simulink model "WDGBrakingLogic_Harness_SLDV"  (R2024a)
settings: Solver=FixedStepDiscrete  StartTime=0  StopTime=0.5  FixedStep=0.10000000000000001  RelTol=1e-3  EnableMultiTasking=on
Description:
  | Test harness for SLDV generated test cases.
settings Model: DataDictionary=DD_WDGBrakingLogic.sldd  EnableAccessToBaseWorkspace=off  Creator=The MathWorks, Inc.  LastModifiedBy=The MathWorks, Inc.
settings SolverCC: MaxZcPerStep=1
settings DataIOCC: LimitDataPoints=on
settings OptimizationCC: BlockReduction=off  DefaultParameterBehavior=Inlined  UseDivisionForNetSlopeComputation=on  GainParamInheritBuiltInType=on  UseFloatMulNetSlope=on  InlineInvariantSignals=on  ExpressionFolding=off  BitwiseOrLogicalOp=Bitwise operator  PassReuseOutputArgsAs=Individual arguments  InitFltsAndDblsToZero=on  EfficientFloat2IntCast=on  LifeSpan=inf  MaxStackSize=inf  OptimizeBlockOrder=speed  DifferentSizesBufferReuse=on  EfficientTunableParamExpr=on
settings DebuggingCC: SignalInfNanChecking=error  SignalRangeChecking=error  ReadBeforeWriteMsg=EnableAllAsError  WriteAfterWriteMsg=EnableAllAsError  WriteAfterReadMsg=EnableAllAsError  AlgebraicLoopMsg=error  ArtificialAlgebraicLoopMsg=error  SaveWithDisabledLinksMsg=error  SaveWithParameterizedLinksMsg=error  BlockPriorityViolationMsg=error  SolverPrmCheckMsg=error  InheritedTsInSrcMsg=none  SingleTaskRateTransMsg=error  TasksWithSamePriorityMsg=error  SigSpecEnsureSampleTimeMsg=error  CheckMatrixSingularityMsg=error  IntegerOverflowMsg=error  ParameterUnderflowMsg=error  ParameterPrecisionLossMsg=error  ParameterTunabilityLossMsg=error  UnderSpecifiedDataTypeMsg=error  UnnecessaryDatatypeConvMsg=warning  VectorMatrixConversionMsg=error  SignalLabelMismatchMsg=error  UnconnectedInputMsg=error  UnconnectedOutputMsg=error  UnconnectedLineMsg=error  SFcnCompatibilityMsg=error  UniqueDataStoreMsg=error  BusObjectLabelMismatch=error  RootOutportRequireBusObject=error  AssertControl=DisableAll  AllowSymbolicDim=off  ModelReferenceIOMismatchMessage=error  UnknownTsInhSupMsg=error  ModelReferenceDataLoggingMessage=error  ModelReferenceSymbolNameMessage=none  StateNameClashWarn=warning  PregeneratedLibrarySubsystemCodeDiagnostic=none  StrictBusMsg=ErrorOnBusTreatedAsVector  NonBusSignalsTreatedAsBus=error  SFInvalidInputDataAccessInChartInitDiag=error  SFTransitionOutsideNaturalParentDiag=error  SFUnreachableExecutionPathDiag=error  SFUndirectedBroadcastEventsDiag=error  SFTransitionActionBeforeConditionDiag=error  SFTemporalDelaySmallerThanSampleTimeDiag=error  SFSelfTransitionDiag=error  SFExecutionAtInitializationDiag=error  IntegerSaturationMsg=error  ArithmeticOperatorsInVariantConditions=warning
settings HardwareCC: ProdLongLongMode=on
settings ModelReferenceCC: EnableRefExpFcnMdlSchedulingChecks=on  PropagateSignalLabelsOutOfModel=off
settings SFSimCC: CompileTimeRecursionLimit=0  EnableRuntimeRecursion=off  MATLABDynamicMemAlloc=off  CustomCodeUndefinedFunction=UseInterfaceOnly
settings RTWCC: Description=Embedded Coder  SystemTargetFile=ert.tlc  GenCodeOnly=on  TemplateMakefile=ert_default_tmf  GenerateReport=on  BuildConfiguration=Faster Runs  IncludeHyperlinkInReport=on  LaunchReport=on  GenerateTraceInfo=on  GenerateTraceReport=on  GenerateTraceReportSl=on  GenerateTraceReportSf=on  GenerateTraceReportEml=on  GenerateCodeMetricsReport=on  GPUComputeCapability=3.5  DLArmComputeVersion=19.05
settings CodeAppCC: ForceParamTrailComments=on  IgnoreCustomStorageClasses=off  MATLABFcnDesc=on  MangleLength=4  StateflowObjectComments=on  ReqsInCode=on
settings ERTTargetCC: TargetLangStandard=C99 (ISO)  UtilityFuncGeneration=Shared location  GenerateSampleERTMain=on  IncludeMdlTerminateFcn=off  CombineSignalStateStructs=on  SuppressErrorStatus=on  SupportAbsoluteTime=off  SupportNonFinite=off  ParenthesesLevel=Maximum  CastingMode=Standards  GenerateSharedConstants=off  InlinedParameterPlacement=NonHierarchical  ERTCustomFileTemplate=example_file_process.tlc  PreserveExpressionOrder=on  EnableSignedLeftShifts=off  EnableSignedRightShifts=off
settings ConfigComp: CovScope=ReferencedModels  CovIncludeTopModel=off  CovMetricSettings=dcmobe  CovHTMLOptions=-aTS=1 -bRG=1 -bTC=0 -hTR=0 -nFC=0 -scm=1 -bcm=1

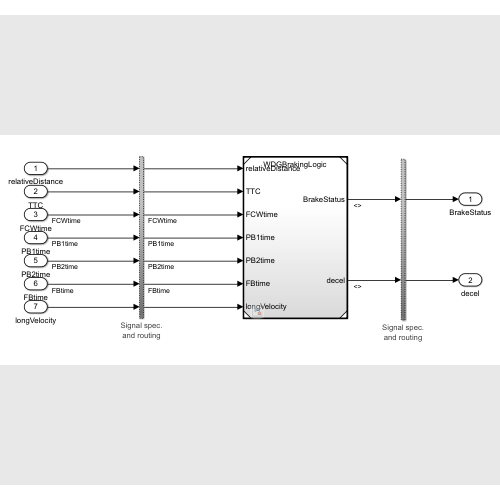
[thumbnail: Simulink's stored preview of the top-level diagram]
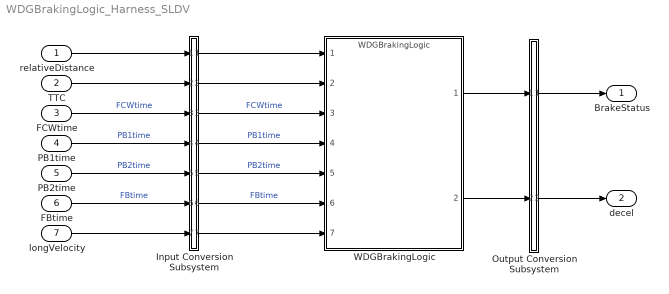
== system WDGBrakingLogic_Harness_SLDV ==
  relativeDistance : Inport  OutDataTypeStr=double  PortDimensions=[1]  SampleTime=0.1  Interpolate=off
  TTC : Inport  Port=2  OutDataTypeStr=double  PortDimensions=[1]  SampleTime=0.1  Interpolate=off
  FCWtime : Inport  Port=3  OutDataTypeStr=double  PortDimensions=[1]  SampleTime=0.1  Interpolate=off
  PB1time : Inport  Port=4  OutDataTypeStr=double  PortDimensions=[1]  SampleTime=0.1  Interpolate=off
  PB2time : Inport  Port=5  OutDataTypeStr=double  PortDimensions=[1]  SampleTime=0.1  Interpolate=off
  FBtime : Inport  Port=6  OutDataTypeStr=double  PortDimensions=[1]  SampleTime=0.1  Interpolate=off
  longVelocity : Inport  Port=7  OutDataTypeStr=double  PortDimensions=[1]  SampleTime=0.1  Interpolate=off
  Input Conversion Subsystem : Subsystem  Tag=__SLT_ICS__  Description=|
      | Signal spec.
      | and routing
      settings: AttributesFormatString=%<Description>
  Output Conversion Subsystem : Subsystem  Tag=__SLT_OCS__  Description=|
      | Signal spec.
      | and routing
      settings: AttributesFormatString=%<Description>
  WDGBrakingLogic : ModelReference  ModelNameDialog=WDGBrakingLogic  SimulationMode=Normal  ModelReferenceVersion=7.0
  BrakeStatus : Outport
  decel : Outport  Port=2
  wires:
  relativeDistance/1 -> Input Conversion Subsystem/1(Inport_1)
  TTC/1 -> Input Conversion Subsystem/2(Inport_2)
  FCWtime/1 -> Input Conversion Subsystem/3(Inport_3)  "FCWtime"
  PB1time/1 -> Input Conversion Subsystem/4(Inport_4)  "PB1time"
  PB2time/1 -> Input Conversion Subsystem/5(Inport_5)  "PB2time"
  FBtime/1 -> Input Conversion Subsystem/6(Inport_6)  "FBtime"
  longVelocity/1 -> Input Conversion Subsystem/7(Inport_7)
  Output Conversion Subsystem/1(Outport_1) -> BrakeStatus/1
  Output Conversion Subsystem/2(Outport_2) -> decel/1
  Input Conversion Subsystem/1(Outport_1) -> WDGBrakingLogic/1
  Input Conversion Subsystem/2(Outport_2) -> WDGBrakingLogic/2
  Input Conversion Subsystem/3(Outport_3) -> WDGBrakingLogic/3  "FCWtime"
  Input Conversion Subsystem/4(Outport_4) -> WDGBrakingLogic/4  "PB1time"
  Input Conversion Subsystem/5(Outport_5) -> WDGBrakingLogic/5  "PB2time"
  Input Conversion Subsystem/6(Outport_6) -> WDGBrakingLogic/6  "FBtime"
  Input Conversion Subsystem/7(Outport_7) -> WDGBrakingLogic/7
  WDGBrakingLogic/1 -> Output Conversion Subsystem/1(Inport_1)
  WDGBrakingLogic/2 -> Output Conversion Subsystem/2(Inport_2)

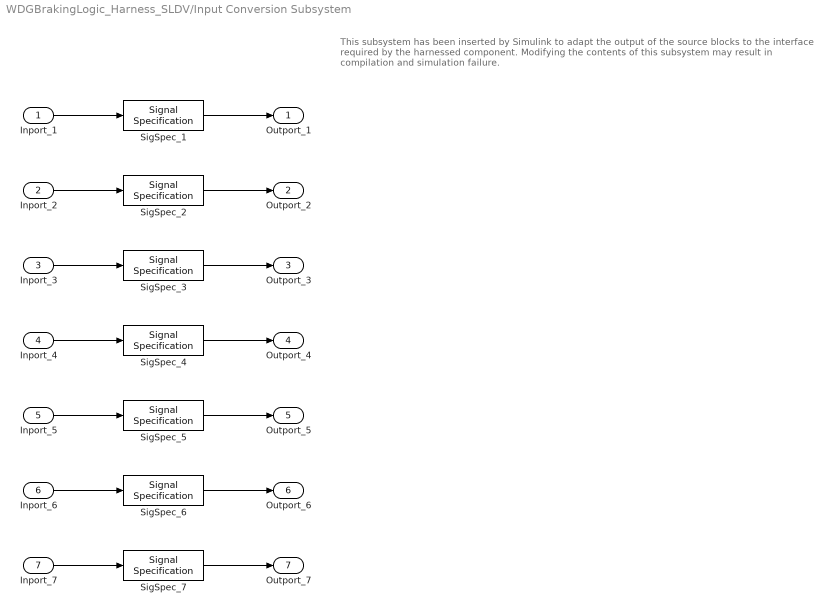
== system WDGBrakingLogic_Harness_SLDV/Input Conversion Subsystem ==
  note: This subsystem has been inserted by Simulink to adapt the output of the source blocks to the interface required by the harnessed component.
      |  Modifying the contents of this subsystem may result in compilation and simulation failure.
  Inport_1 : Inport
  Inport_2 : Inport  Port=2
  Inport_3 : Inport  Port=3
  Inport_4 : Inport  Port=4
  Inport_5 : Inport  Port=5
  Inport_6 : Inport  Port=6
  Inport_7 : Inport  Port=7
  SigSpec_1 : SignalSpecification  OutDataTypeStr=double  Unit=m  Dimensions=[1]  SampleTime=0.1
  SigSpec_{2..6} (5 alike) : SignalSpecification  OutDataTypeStr=double  Unit=s  Dimensions=[1]  SampleTime=0.1
  SigSpec_7 : SignalSpecification  OutDataTypeStr=double  Unit=m/s  Dimensions=[1]  SampleTime=0.1
  Outport_1 : Outport
  Outport_2 : Outport  Port=2
  Outport_3 : Outport  Port=3
  Outport_4 : Outport  Port=4
  Outport_5 : Outport  Port=5
  Outport_6 : Outport  Port=6
  Outport_7 : Outport  Port=7
  wires:
  SigSpec_1/1 -> Outport_1/1
  Inport_1/1 -> SigSpec_1/1
  SigSpec_2/1 -> Outport_2/1
  Inport_2/1 -> SigSpec_2/1
  SigSpec_3/1 -> Outport_3/1
  Inport_3/1 -> SigSpec_3/1
  SigSpec_4/1 -> Outport_4/1
  Inport_4/1 -> SigSpec_4/1
  SigSpec_5/1 -> Outport_5/1
  Inport_5/1 -> SigSpec_5/1
  SigSpec_6/1 -> Outport_6/1
  Inport_6/1 -> SigSpec_6/1
  SigSpec_7/1 -> Outport_7/1
  Inport_7/1 -> SigSpec_7/1

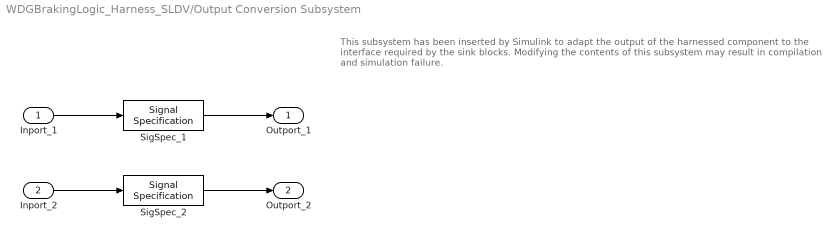
== system WDGBrakingLogic_Harness_SLDV/Output Conversion Subsystem ==
  note: This subsystem has been inserted by Simulink to adapt the output of the harnessed component to the interface required by the sink blocks.
      |  Modifying the contents of this subsystem may result in compilation and simulation failure.
  Inport_1 : Inport
  Inport_2 : Inport  Port=2
  SigSpec_1 : SignalSpecification  OutDataTypeStr=Enum: BrStatus  Dimensions=[1]  SampleTime=0.1
  SigSpec_2 : SignalSpecification  OutDataTypeStr=double  Unit=m/s^2  Dimensions=[1]  SampleTime=0.1
  Outport_1 : Outport
  Outport_2 : Outport  Port=2
  wires:
  Inport_1/1 -> SigSpec_1/1
  SigSpec_1/1 -> Outport_1/1
  Inport_2/1 -> SigSpec_2/1
  SigSpec_2/1 -> Outport_2/1
